simulink model "camera_model_2019b"  (R2019b)
settings: Solver=VariableStepAuto  StartTime=0.0  StopTime=10.0  RelTol=1e-3
values from neighbouring files (symbols this model uses):
  ang = [pi/2 pi/2 0]    [init.m]
  d = C - O    [camera.m]    (also in init.m)
  f = 0.015    [camera.m]    (also in init.m = 0.05)
  p = [4.6; 0.25; 1.8]    [camera.m]    (also in init.m = [1.0; 0.15; 0.8])
settings Model: Creator=antonio  LastModifiedBy=antonio

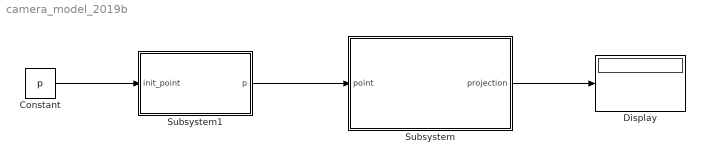
== system camera_model_2019b ==
  Constant : Constant  Value=p
  Display : Display
  Subsystem : Subsystem
  Subsystem1 : Subsystem
  wires:
  Subsystem/1(projection) -> Display/1
  Constant/1 -> Subsystem1/1(init_point)
  Subsystem1/1(p) -> Subsystem/1(point)

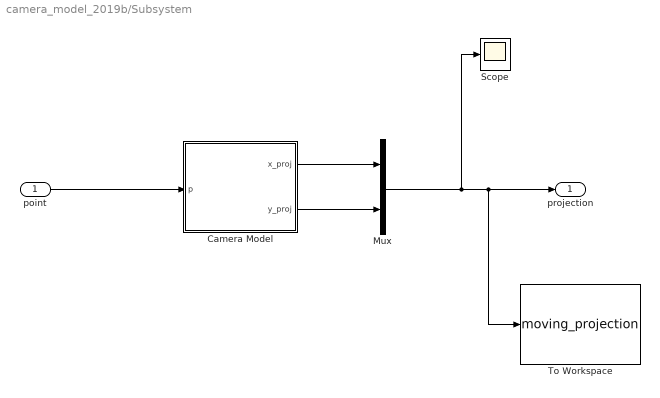
== system camera_model_2019b/Subsystem ==
  point : Inport
  Camera Model : MATLAB Function  TreatAsAtomicUnit=on
  Mux : Mux  Inputs=2
  Scope : Scope
  To Workspace : ToWorkspace  VariableName=moving_projection  SampleTime=0.1
  projection : Outport
  wires:
  Camera Model/1(x_proj) -> Mux/1
  Camera Model/2(y_proj) -> Mux/2
  Mux/1 -> Scope/1, projection/1, To Workspace/1
  point/1 -> Camera Model/1(p)

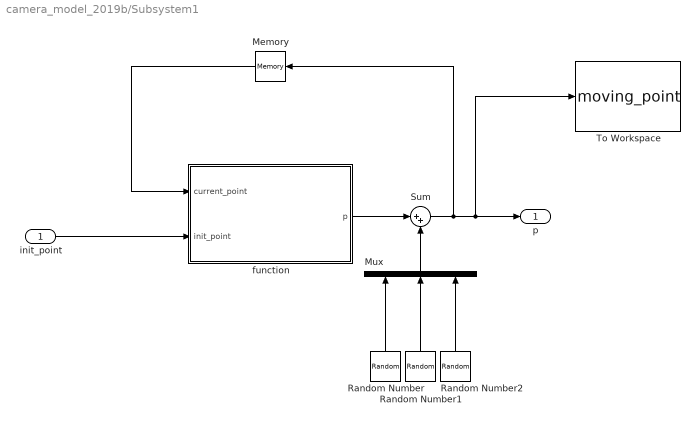
== system camera_model_2019b/Subsystem1 ==
  init_point : Inport
  Memory : Memory  InitialCondition=zeros(3, 1)
  Mux : Mux  Inputs=3
  Random Number : RandomNumber  Variance=0.002  SampleTime=0.3
  Random Number1 : RandomNumber  Variance=0.002  Seed=2  SampleTime=0.3
  Random Number2 : RandomNumber  Variance=0.002  Seed=5  SampleTime=0.3
  Sum : Sum  Inputs=|++
  To Workspace : ToWorkspace  VariableName=moving_point  SampleTime=-1
  function : MATLAB Function  TreatAsAtomicUnit=on
  p : Outport
  wires:
  Memory/1 -> function/1(current_point)
  init_point/1 -> function/2(init_point)
  function/1(p) -> Sum/1
  Sum/1 -> Memory/1, To Workspace/1, p/1
  Mux/1 -> Sum/2
  Random Number/1 -> Mux/1
  Random Number1/1 -> Mux/2
  Random Number2/1 -> Mux/3

== matlab function camera_model_2019b/Subsystem1/function ==
  data: current_point input; init_point input; p output
function p = fcn(current_point, init_point)

if current_point == zeros(3,1)
    p = init_point;
else
    p = current_point;
end

== matlab function camera_model_2019b/Subsystem/Camera Model ==
  data: p input; x_proj output; y_proj output; ang parameter; d parameter; f parameter
function [x_proj,y_proj] = proj(p, ang, d, f)

Twc = [rot(ang(1),ang(2),ang(3))   d;
                zeros(1,3)         1];

p_cam = Twc^-1 * [p;1];   % point's position in camera frame

P = diag([f,f,1]) * [eye(3), zeros(3,1)]; % camera projection matrix

p_tilde = P*p_cam;       
x_proj = -p_tilde(1)/p(3);
y_proj = p_tilde(2)/p(3);

end
